simulink model "AE_315_W2_RLC_circuit_charge"  (R2022b)
settings: Solver=VariableStepAuto  StartTime=0.0  StopTime=1e-3  RelTol=1e-3
settings Model: Creator=SoftLaptop  LastModifiedBy=SoftLaptop

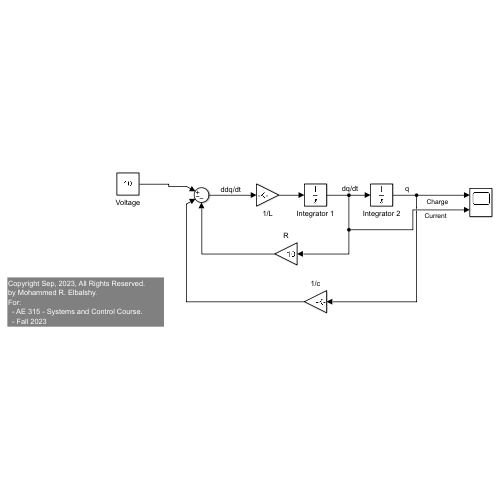
[thumbnail: Simulink's stored preview of the top-level diagram]
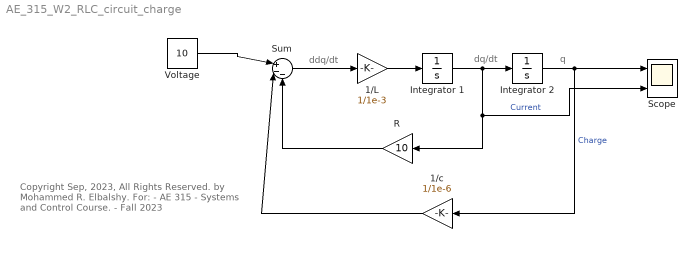
== system AE_315_W2_RLC_circuit_charge ==
  note: ddq/dt
  note: q
  note: dq/dt
  note: Copyright Sep, 2023, All Rights Reserved.
      | by Mohammed R. Elbalshy.
      | For:
      | - AE 315 - Systems and Control Course.
      | - Fall 2023
  1/L : Gain  Gain=1/1e-3
  1/c : Gain  Gain=1/1e-6
  Integrator 1 : Integrator  InitialCondition=1
  Integrator 2 : Integrator
  R : Gain  Gain=10
  Scope : Scope  NumInputPorts=2
  Sum : Sum  Inputs=|+--
  Voltage : Constant  Value=10
  wires:
  Integrator 1/1 -> Scope/2, R/1, Integrator 2/1  "Current"
  1/L/1 -> Integrator 1/1
  Voltage/1 -> Sum/1
  Integrator 2/1 -> Scope/1, 1/c/1  "Charge"
  Sum/1 -> 1/L/1
  R/1 -> Sum/3
  1/c/1 -> Sum/2
